simulink model "lo_values_test_v11"  (R2012b)
settings: Solver=ode45  StartTime=0.0  StopTime=100000  RelTol=1e-3
values from neighbouring files (symbols this model uses):
  Fs = 640e6    (= 640000000)    [filter_coefficients.m]    (also in filter_design.m; filter_design_getting_order.m)
undefined symbols (not defined in the file or in its folder): get, sided, Two
undefined symbols (not defined in the file): A_cos, A_sin, B_cos, B_sin, C_cos, C_sin, casper_coef, coef, D_cos, D_sin
libraries: xbsIndex_r4 x1768, dspsnks4 x10, casper_library_misc x9, xps_library x2, simulink x1
(part 6 of 17)

== system lo_values_test_v11/dec_fir2/fir_dbl_col38 ==
  real1 : Inport
  imag1 : Inport  Port=2
  real_back1 : Inport  Port=3
  imag_back1 : Inport  Port=4
  fir_dbl_tap1 : Subsystem  AncestorBlock=casper_library_downconverter/fir_dbl_tap  mask(fir_dbl_tap){factor=0.011867, add_latency=add_latency, mult_latency=mult_latency, coeff_bit_width=coeff_bit_width, coeff_bin_pt=coeff_bin_pt}
      mask prompts: add_latency "Add latency"; mult_latency "Mult latency"; coeff_bit_width "Coefficient bit width"; coeff_bin_pt "Coefficient binary point"
      mask init: same as lo_values_test_v11/dec_fir/fir_dbl_col1/fir_dbl_tap1
      mask Help: eval('xlWeb(''http://casper.berkeley.edu/wiki/Fir_dbl_tap'')')
  real_out1 : Outport
  imag_out1 : Outport  Port=2
  real_back_out1 : Outport  Port=3
  imag_back_out1 : Outport  Port=4
  real_sum : Outport  Port=5
  imag_sum : Outport  Port=6
  wires:
  real1/1 -> fir_dbl_tap1/1(a)
  imag1/1 -> fir_dbl_tap1/2(b)
  real_back1/1 -> fir_dbl_tap1/3(c)
  imag_back1/1 -> fir_dbl_tap1/4(d)
  fir_dbl_tap1/1(a_out) -> real_out1/1
  fir_dbl_tap1/2(b_out) -> imag_out1/1
  fir_dbl_tap1/3(c_out) -> real_back_out1/1
  fir_dbl_tap1/4(d_out) -> imag_back_out1/1
  fir_dbl_tap1/5(real) -> real_sum/1
  fir_dbl_tap1/6(imag) -> imag_sum/1

== system lo_values_test_v11/dec_fir2/fir_dbl_col39 ==
  real1 : Inport
  imag1 : Inport  Port=2
  real_back1 : Inport  Port=3
  imag_back1 : Inport  Port=4
  fir_dbl_tap1 : Subsystem  AncestorBlock=casper_library_downconverter/fir_dbl_tap  mask(fir_dbl_tap){factor=0.012277, add_latency=add_latency, mult_latency=mult_latency, coeff_bit_width=coeff_bit_width, coeff_bin_pt=coeff_bin_pt}
      mask prompts: add_latency "Add latency"; mult_latency "Mult latency"; coeff_bit_width "Coefficient bit width"; coeff_bin_pt "Coefficient binary point"
      mask init: same as lo_values_test_v11/dec_fir/fir_dbl_col1/fir_dbl_tap1
      mask Help: eval('xlWeb(''http://casper.berkeley.edu/wiki/Fir_dbl_tap'')')
  real_out1 : Outport
  imag_out1 : Outport  Port=2
  real_back_out1 : Outport  Port=3
  imag_back_out1 : Outport  Port=4
  real_sum : Outport  Port=5
  imag_sum : Outport  Port=6
  wires:
  real1/1 -> fir_dbl_tap1/1(a)
  imag1/1 -> fir_dbl_tap1/2(b)
  real_back1/1 -> fir_dbl_tap1/3(c)
  imag_back1/1 -> fir_dbl_tap1/4(d)
  fir_dbl_tap1/1(a_out) -> real_out1/1
  fir_dbl_tap1/2(b_out) -> imag_out1/1
  fir_dbl_tap1/3(c_out) -> real_back_out1/1
  fir_dbl_tap1/4(d_out) -> imag_back_out1/1
  fir_dbl_tap1/5(real) -> real_sum/1
  fir_dbl_tap1/6(imag) -> imag_sum/1

== system lo_values_test_v11/dec_fir2/fir_dbl_col4 ==
  real1 : Inport
  imag1 : Inport  Port=2
  real_back1 : Inport  Port=3
  imag_back1 : Inport  Port=4
  fir_dbl_tap1 : Subsystem  AncestorBlock=casper_library_downconverter/fir_dbl_tap  mask(fir_dbl_tap){factor=0.00035551, add_latency=add_latency, mult_latency=mult_latency, coeff_bit_width=coeff_bit_width, coeff_bin_pt=coeff_bin_pt}
      mask prompts: add_latency "Add latency"; mult_latency "Mult latency"; coeff_bit_width "Coefficient bit width"; coeff_bin_pt "Coefficient binary point"
      mask init: same as lo_values_test_v11/dec_fir/fir_dbl_col1/fir_dbl_tap1
      mask Help: eval('xlWeb(''http://casper.berkeley.edu/wiki/Fir_dbl_tap'')')
  real_out1 : Outport
  imag_out1 : Outport  Port=2
  real_back_out1 : Outport  Port=3
  imag_back_out1 : Outport  Port=4
  real_sum : Outport  Port=5
  imag_sum : Outport  Port=6
  wires:
  real1/1 -> fir_dbl_tap1/1(a)
  imag1/1 -> fir_dbl_tap1/2(b)
  real_back1/1 -> fir_dbl_tap1/3(c)
  imag_back1/1 -> fir_dbl_tap1/4(d)
  fir_dbl_tap1/1(a_out) -> real_out1/1
  fir_dbl_tap1/2(b_out) -> imag_out1/1
  fir_dbl_tap1/3(c_out) -> real_back_out1/1
  fir_dbl_tap1/4(d_out) -> imag_back_out1/1
  fir_dbl_tap1/5(real) -> real_sum/1
  fir_dbl_tap1/6(imag) -> imag_sum/1

== system lo_values_test_v11/dec_fir2/fir_dbl_col40 ==
  real1 : Inport
  imag1 : Inport  Port=2
  real_back1 : Inport  Port=3
  imag_back1 : Inport  Port=4
  fir_dbl_tap1 : Subsystem  AncestorBlock=casper_library_downconverter/fir_dbl_tap  mask(fir_dbl_tap){factor=0.012666, add_latency=add_latency, mult_latency=mult_latency, coeff_bit_width=coeff_bit_width, coeff_bin_pt=coeff_bin_pt}
      mask prompts: add_latency "Add latency"; mult_latency "Mult latency"; coeff_bit_width "Coefficient bit width"; coeff_bin_pt "Coefficient binary point"
      mask init: same as lo_values_test_v11/dec_fir/fir_dbl_col1/fir_dbl_tap1
      mask Help: eval('xlWeb(''http://casper.berkeley.edu/wiki/Fir_dbl_tap'')')
  real_out1 : Outport
  imag_out1 : Outport  Port=2
  real_back_out1 : Outport  Port=3
  imag_back_out1 : Outport  Port=4
  real_sum : Outport  Port=5
  imag_sum : Outport  Port=6
  wires:
  real1/1 -> fir_dbl_tap1/1(a)
  imag1/1 -> fir_dbl_tap1/2(b)
  real_back1/1 -> fir_dbl_tap1/3(c)
  imag_back1/1 -> fir_dbl_tap1/4(d)
  fir_dbl_tap1/1(a_out) -> real_out1/1
  fir_dbl_tap1/2(b_out) -> imag_out1/1
  fir_dbl_tap1/3(c_out) -> real_back_out1/1
  fir_dbl_tap1/4(d_out) -> imag_back_out1/1
  fir_dbl_tap1/5(real) -> real_sum/1
  fir_dbl_tap1/6(imag) -> imag_sum/1

== system lo_values_test_v11/dec_fir2/fir_dbl_col41 ==
  real1 : Inport
  imag1 : Inport  Port=2
  real_back1 : Inport  Port=3
  imag_back1 : Inport  Port=4
  fir_dbl_tap1 : Subsystem  AncestorBlock=casper_library_downconverter/fir_dbl_tap  mask(fir_dbl_tap){factor=0.013032, add_latency=add_latency, mult_latency=mult_latency, coeff_bit_width=coeff_bit_width, coeff_bin_pt=coeff_bin_pt}
      mask prompts: add_latency "Add latency"; mult_latency "Mult latency"; coeff_bit_width "Coefficient bit width"; coeff_bin_pt "Coefficient binary point"
      mask init: same as lo_values_test_v11/dec_fir/fir_dbl_col1/fir_dbl_tap1
      mask Help: eval('xlWeb(''http://casper.berkeley.edu/wiki/Fir_dbl_tap'')')
  real_out1 : Outport
  imag_out1 : Outport  Port=2
  real_back_out1 : Outport  Port=3
  imag_back_out1 : Outport  Port=4
  real_sum : Outport  Port=5
  imag_sum : Outport  Port=6
  wires:
  real1/1 -> fir_dbl_tap1/1(a)
  imag1/1 -> fir_dbl_tap1/2(b)
  real_back1/1 -> fir_dbl_tap1/3(c)
  imag_back1/1 -> fir_dbl_tap1/4(d)
  fir_dbl_tap1/1(a_out) -> real_out1/1
  fir_dbl_tap1/2(b_out) -> imag_out1/1
  fir_dbl_tap1/3(c_out) -> real_back_out1/1
  fir_dbl_tap1/4(d_out) -> imag_back_out1/1
  fir_dbl_tap1/5(real) -> real_sum/1
  fir_dbl_tap1/6(imag) -> imag_sum/1

== system lo_values_test_v11/dec_fir2/fir_dbl_col42 ==
  real1 : Inport
  imag1 : Inport  Port=2
  real_back1 : Inport  Port=3
  imag_back1 : Inport  Port=4
  fir_dbl_tap1 : Subsystem  AncestorBlock=casper_library_downconverter/fir_dbl_tap  mask(fir_dbl_tap){factor=0.013373, add_latency=add_latency, mult_latency=mult_latency, coeff_bit_width=coeff_bit_width, coeff_bin_pt=coeff_bin_pt}
      mask prompts: add_latency "Add latency"; mult_latency "Mult latency"; coeff_bit_width "Coefficient bit width"; coeff_bin_pt "Coefficient binary point"
      mask init: same as lo_values_test_v11/dec_fir/fir_dbl_col1/fir_dbl_tap1
      mask Help: eval('xlWeb(''http://casper.berkeley.edu/wiki/Fir_dbl_tap'')')
  real_out1 : Outport
  imag_out1 : Outport  Port=2
  real_back_out1 : Outport  Port=3
  imag_back_out1 : Outport  Port=4
  real_sum : Outport  Port=5
  imag_sum : Outport  Port=6
  wires:
  real1/1 -> fir_dbl_tap1/1(a)
  imag1/1 -> fir_dbl_tap1/2(b)
  real_back1/1 -> fir_dbl_tap1/3(c)
  imag_back1/1 -> fir_dbl_tap1/4(d)
  fir_dbl_tap1/1(a_out) -> real_out1/1
  fir_dbl_tap1/2(b_out) -> imag_out1/1
  fir_dbl_tap1/3(c_out) -> real_back_out1/1
  fir_dbl_tap1/4(d_out) -> imag_back_out1/1
  fir_dbl_tap1/5(real) -> real_sum/1
  fir_dbl_tap1/6(imag) -> imag_sum/1

== system lo_values_test_v11/dec_fir2/fir_dbl_col43 ==
  real1 : Inport
  imag1 : Inport  Port=2
  real_back1 : Inport  Port=3
  imag_back1 : Inport  Port=4
  fir_dbl_tap1 : Subsystem  AncestorBlock=casper_library_downconverter/fir_dbl_tap  mask(fir_dbl_tap){factor=0.013686, add_latency=add_latency, mult_latency=mult_latency, coeff_bit_width=coeff_bit_width, coeff_bin_pt=coeff_bin_pt}
      mask prompts: add_latency "Add latency"; mult_latency "Mult latency"; coeff_bit_width "Coefficient bit width"; coeff_bin_pt "Coefficient binary point"
      mask init: same as lo_values_test_v11/dec_fir/fir_dbl_col1/fir_dbl_tap1
      mask Help: eval('xlWeb(''http://casper.berkeley.edu/wiki/Fir_dbl_tap'')')
  real_out1 : Outport
  imag_out1 : Outport  Port=2
  real_back_out1 : Outport  Port=3
  imag_back_out1 : Outport  Port=4
  real_sum : Outport  Port=5
  imag_sum : Outport  Port=6
  wires:
  real1/1 -> fir_dbl_tap1/1(a)
  imag1/1 -> fir_dbl_tap1/2(b)
  real_back1/1 -> fir_dbl_tap1/3(c)
  imag_back1/1 -> fir_dbl_tap1/4(d)
  fir_dbl_tap1/1(a_out) -> real_out1/1
  fir_dbl_tap1/2(b_out) -> imag_out1/1
  fir_dbl_tap1/3(c_out) -> real_back_out1/1
  fir_dbl_tap1/4(d_out) -> imag_back_out1/1
  fir_dbl_tap1/5(real) -> real_sum/1
  fir_dbl_tap1/6(imag) -> imag_sum/1

== system lo_values_test_v11/dec_fir2/fir_dbl_col44 ==
  real1 : Inport
  imag1 : Inport  Port=2
  real_back1 : Inport  Port=3
  imag_back1 : Inport  Port=4
  fir_dbl_tap1 : Subsystem  AncestorBlock=casper_library_downconverter/fir_dbl_tap  mask(fir_dbl_tap){factor=0.01397, add_latency=add_latency, mult_latency=mult_latency, coeff_bit_width=coeff_bit_width, coeff_bin_pt=coeff_bin_pt}
      mask prompts: add_latency "Add latency"; mult_latency "Mult latency"; coeff_bit_width "Coefficient bit width"; coeff_bin_pt "Coefficient binary point"
      mask init: same as lo_values_test_v11/dec_fir/fir_dbl_col1/fir_dbl_tap1
      mask Help: eval('xlWeb(''http://casper.berkeley.edu/wiki/Fir_dbl_tap'')')
  real_out1 : Outport
  imag_out1 : Outport  Port=2
  real_back_out1 : Outport  Port=3
  imag_back_out1 : Outport  Port=4
  real_sum : Outport  Port=5
  imag_sum : Outport  Port=6
  wires:
  real1/1 -> fir_dbl_tap1/1(a)
  imag1/1 -> fir_dbl_tap1/2(b)
  real_back1/1 -> fir_dbl_tap1/3(c)
  imag_back1/1 -> fir_dbl_tap1/4(d)
  fir_dbl_tap1/1(a_out) -> real_out1/1
  fir_dbl_tap1/2(b_out) -> imag_out1/1
  fir_dbl_tap1/3(c_out) -> real_back_out1/1
  fir_dbl_tap1/4(d_out) -> imag_back_out1/1
  fir_dbl_tap1/5(real) -> real_sum/1
  fir_dbl_tap1/6(imag) -> imag_sum/1

== system lo_values_test_v11/dec_fir2/fir_dbl_col45 ==
  real1 : Inport
  imag1 : Inport  Port=2
  real_back1 : Inport  Port=3
  imag_back1 : Inport  Port=4
  fir_dbl_tap1 : Subsystem  AncestorBlock=casper_library_downconverter/fir_dbl_tap  mask(fir_dbl_tap){factor=0.014223, add_latency=add_latency, mult_latency=mult_latency, coeff_bit_width=coeff_bit_width, coeff_bin_pt=coeff_bin_pt}
      mask prompts: add_latency "Add latency"; mult_latency "Mult latency"; coeff_bit_width "Coefficient bit width"; coeff_bin_pt "Coefficient binary point"
      mask init: same as lo_values_test_v11/dec_fir/fir_dbl_col1/fir_dbl_tap1
      mask Help: eval('xlWeb(''http://casper.berkeley.edu/wiki/Fir_dbl_tap'')')
  real_out1 : Outport
  imag_out1 : Outport  Port=2
  real_back_out1 : Outport  Port=3
  imag_back_out1 : Outport  Port=4
  real_sum : Outport  Port=5
  imag_sum : Outport  Port=6
  wires:
  real1/1 -> fir_dbl_tap1/1(a)
  imag1/1 -> fir_dbl_tap1/2(b)
  real_back1/1 -> fir_dbl_tap1/3(c)
  imag_back1/1 -> fir_dbl_tap1/4(d)
  fir_dbl_tap1/1(a_out) -> real_out1/1
  fir_dbl_tap1/2(b_out) -> imag_out1/1
  fir_dbl_tap1/3(c_out) -> real_back_out1/1
  fir_dbl_tap1/4(d_out) -> imag_back_out1/1
  fir_dbl_tap1/5(real) -> real_sum/1
  fir_dbl_tap1/6(imag) -> imag_sum/1

== system lo_values_test_v11/dec_fir2/fir_dbl_col46 ==
  real1 : Inport
  imag1 : Inport  Port=2
  real_back1 : Inport  Port=3
  imag_back1 : Inport  Port=4
  fir_dbl_tap1 : Subsystem  AncestorBlock=casper_library_downconverter/fir_dbl_tap  mask(fir_dbl_tap){factor=0.014442, add_latency=add_latency, mult_latency=mult_latency, coeff_bit_width=coeff_bit_width, coeff_bin_pt=coeff_bin_pt}
      mask prompts: add_latency "Add latency"; mult_latency "Mult latency"; coeff_bit_width "Coefficient bit width"; coeff_bin_pt "Coefficient binary point"
      mask init: same as lo_values_test_v11/dec_fir/fir_dbl_col1/fir_dbl_tap1
      mask Help: eval('xlWeb(''http://casper.berkeley.edu/wiki/Fir_dbl_tap'')')
  real_out1 : Outport
  imag_out1 : Outport  Port=2
  real_back_out1 : Outport  Port=3
  imag_back_out1 : Outport  Port=4
  real_sum : Outport  Port=5
  imag_sum : Outport  Port=6
  wires:
  real1/1 -> fir_dbl_tap1/1(a)
  imag1/1 -> fir_dbl_tap1/2(b)
  real_back1/1 -> fir_dbl_tap1/3(c)
  imag_back1/1 -> fir_dbl_tap1/4(d)
  fir_dbl_tap1/1(a_out) -> real_out1/1
  fir_dbl_tap1/2(b_out) -> imag_out1/1
  fir_dbl_tap1/3(c_out) -> real_back_out1/1
  fir_dbl_tap1/4(d_out) -> imag_back_out1/1
  fir_dbl_tap1/5(real) -> real_sum/1
  fir_dbl_tap1/6(imag) -> imag_sum/1

== system lo_values_test_v11/dec_fir2/fir_dbl_col47 ==
  real1 : Inport
  imag1 : Inport  Port=2
  real_back1 : Inport  Port=3
  imag_back1 : Inport  Port=4
  fir_dbl_tap1 : Subsystem  AncestorBlock=casper_library_downconverter/fir_dbl_tap  mask(fir_dbl_tap){factor=0.014628, add_latency=add_latency, mult_latency=mult_latency, coeff_bit_width=coeff_bit_width, coeff_bin_pt=coeff_bin_pt}
      mask prompts: add_latency "Add latency"; mult_latency "Mult latency"; coeff_bit_width "Coefficient bit width"; coeff_bin_pt "Coefficient binary point"
      mask init: same as lo_values_test_v11/dec_fir/fir_dbl_col1/fir_dbl_tap1
      mask Help: eval('xlWeb(''http://casper.berkeley.edu/wiki/Fir_dbl_tap'')')
  real_out1 : Outport
  imag_out1 : Outport  Port=2
  real_back_out1 : Outport  Port=3
  imag_back_out1 : Outport  Port=4
  real_sum : Outport  Port=5
  imag_sum : Outport  Port=6
  wires:
  real1/1 -> fir_dbl_tap1/1(a)
  imag1/1 -> fir_dbl_tap1/2(b)
  real_back1/1 -> fir_dbl_tap1/3(c)
  imag_back1/1 -> fir_dbl_tap1/4(d)
  fir_dbl_tap1/1(a_out) -> real_out1/1
  fir_dbl_tap1/2(b_out) -> imag_out1/1
  fir_dbl_tap1/3(c_out) -> real_back_out1/1
  fir_dbl_tap1/4(d_out) -> imag_back_out1/1
  fir_dbl_tap1/5(real) -> real_sum/1
  fir_dbl_tap1/6(imag) -> imag_sum/1

== system lo_values_test_v11/dec_fir2/fir_dbl_col48 ==
  real1 : Inport
  imag1 : Inport  Port=2
  real_back1 : Inport  Port=3
  imag_back1 : Inport  Port=4
  fir_dbl_tap1 : Subsystem  AncestorBlock=casper_library_downconverter/fir_dbl_tap  mask(fir_dbl_tap){factor=0.014778, add_latency=add_latency, mult_latency=mult_latency, coeff_bit_width=coeff_bit_width, coeff_bin_pt=coeff_bin_pt}
      mask prompts: add_latency "Add latency"; mult_latency "Mult latency"; coeff_bit_width "Coefficient bit width"; coeff_bin_pt "Coefficient binary point"
      mask init: same as lo_values_test_v11/dec_fir/fir_dbl_col1/fir_dbl_tap1
      mask Help: eval('xlWeb(''http://casper.berkeley.edu/wiki/Fir_dbl_tap'')')
  real_out1 : Outport
  imag_out1 : Outport  Port=2
  real_back_out1 : Outport  Port=3
  imag_back_out1 : Outport  Port=4
  real_sum : Outport  Port=5
  imag_sum : Outport  Port=6
  wires:
  real1/1 -> fir_dbl_tap1/1(a)
  imag1/1 -> fir_dbl_tap1/2(b)
  real_back1/1 -> fir_dbl_tap1/3(c)
  imag_back1/1 -> fir_dbl_tap1/4(d)
  fir_dbl_tap1/1(a_out) -> real_out1/1
  fir_dbl_tap1/2(b_out) -> imag_out1/1
  fir_dbl_tap1/3(c_out) -> real_back_out1/1
  fir_dbl_tap1/4(d_out) -> imag_back_out1/1
  fir_dbl_tap1/5(real) -> real_sum/1
  fir_dbl_tap1/6(imag) -> imag_sum/1

== system lo_values_test_v11/dec_fir2/fir_dbl_col49 ==
  real1 : Inport
  imag1 : Inport  Port=2
  real_back1 : Inport  Port=3
  imag_back1 : Inport  Port=4
  fir_dbl_tap1 : Subsystem  AncestorBlock=casper_library_downconverter/fir_dbl_tap  mask(fir_dbl_tap){factor=0.014891, add_latency=add_latency, mult_latency=mult_latency, coeff_bit_width=coeff_bit_width, coeff_bin_pt=coeff_bin_pt}
      mask prompts: add_latency "Add latency"; mult_latency "Mult latency"; coeff_bit_width "Coefficient bit width"; coeff_bin_pt "Coefficient binary point"
      mask init: same as lo_values_test_v11/dec_fir/fir_dbl_col1/fir_dbl_tap1
      mask Help: eval('xlWeb(''http://casper.berkeley.edu/wiki/Fir_dbl_tap'')')
  real_out1 : Outport
  imag_out1 : Outport  Port=2
  real_back_out1 : Outport  Port=3
  imag_back_out1 : Outport  Port=4
  real_sum : Outport  Port=5
  imag_sum : Outport  Port=6
  wires:
  real1/1 -> fir_dbl_tap1/1(a)
  imag1/1 -> fir_dbl_tap1/2(b)
  real_back1/1 -> fir_dbl_tap1/3(c)
  imag_back1/1 -> fir_dbl_tap1/4(d)
  fir_dbl_tap1/1(a_out) -> real_out1/1
  fir_dbl_tap1/2(b_out) -> imag_out1/1
  fir_dbl_tap1/3(c_out) -> real_back_out1/1
  fir_dbl_tap1/4(d_out) -> imag_back_out1/1
  fir_dbl_tap1/5(real) -> real_sum/1
  fir_dbl_tap1/6(imag) -> imag_sum/1

== system lo_values_test_v11/dec_fir2/fir_dbl_col5 ==
  real1 : Inport
  imag1 : Inport  Port=2
  real_back1 : Inport  Port=3
  imag_back1 : Inport  Port=4
  fir_dbl_tap1 : Subsystem  AncestorBlock=casper_library_downconverter/fir_dbl_tap  mask(fir_dbl_tap){factor=0.00044384, add_latency=add_latency, mult_latency=mult_latency, coeff_bit_width=coeff_bit_width, coeff_bin_pt=coeff_bin_pt}
      mask prompts: add_latency "Add latency"; mult_latency "Mult latency"; coeff_bit_width "Coefficient bit width"; coeff_bin_pt "Coefficient binary point"
      mask init: same as lo_values_test_v11/dec_fir/fir_dbl_col1/fir_dbl_tap1
      mask Help: eval('xlWeb(''http://casper.berkeley.edu/wiki/Fir_dbl_tap'')')
  real_out1 : Outport
  imag_out1 : Outport  Port=2
  real_back_out1 : Outport  Port=3
  imag_back_out1 : Outport  Port=4
  real_sum : Outport  Port=5
  imag_sum : Outport  Port=6
  wires:
  real1/1 -> fir_dbl_tap1/1(a)
  imag1/1 -> fir_dbl_tap1/2(b)
  real_back1/1 -> fir_dbl_tap1/3(c)
  imag_back1/1 -> fir_dbl_tap1/4(d)
  fir_dbl_tap1/1(a_out) -> real_out1/1
  fir_dbl_tap1/2(b_out) -> imag_out1/1
  fir_dbl_tap1/3(c_out) -> real_back_out1/1
  fir_dbl_tap1/4(d_out) -> imag_back_out1/1
  fir_dbl_tap1/5(real) -> real_sum/1
  fir_dbl_tap1/6(imag) -> imag_sum/1

== system lo_values_test_v11/dec_fir2/fir_dbl_col50 ==
  real1 : Inport
  imag1 : Inport  Port=2
  real_back1 : Inport  Port=3
  imag_back1 : Inport  Port=4
  fir_dbl_tap1 : Subsystem  AncestorBlock=casper_library_downconverter/fir_dbl_tap  mask(fir_dbl_tap){factor=0.014967, add_latency=add_latency, mult_latency=mult_latency, coeff_bit_width=coeff_bit_width, coeff_bin_pt=coeff_bin_pt}
      mask prompts: add_latency "Add latency"; mult_latency "Mult latency"; coeff_bit_width "Coefficient bit width"; coeff_bin_pt "Coefficient binary point"
      mask init: same as lo_values_test_v11/dec_fir/fir_dbl_col1/fir_dbl_tap1
      mask Help: eval('xlWeb(''http://casper.berkeley.edu/wiki/Fir_dbl_tap'')')
  real_out1 : Outport
  imag_out1 : Outport  Port=2
  real_back_out1 : Outport  Port=3
  imag_back_out1 : Outport  Port=4
  real_sum : Outport  Port=5
  imag_sum : Outport  Port=6
  wires:
  real1/1 -> fir_dbl_tap1/1(a)
  imag1/1 -> fir_dbl_tap1/2(b)
  real_back1/1 -> fir_dbl_tap1/3(c)
  imag_back1/1 -> fir_dbl_tap1/4(d)
  fir_dbl_tap1/1(a_out) -> real_out1/1
  fir_dbl_tap1/2(b_out) -> imag_out1/1
  fir_dbl_tap1/3(c_out) -> real_back_out1/1
  fir_dbl_tap1/4(d_out) -> imag_back_out1/1
  fir_dbl_tap1/5(real) -> real_sum/1
  fir_dbl_tap1/6(imag) -> imag_sum/1

== system lo_values_test_v11/dec_fir2/fir_dbl_col51 ==
  real1 : Inport
  imag1 : Inport  Port=2
  real_back1 : Inport  Port=3
  imag_back1 : Inport  Port=4
  fir_dbl_tap1 : Subsystem  AncestorBlock=casper_library_downconverter/fir_dbl_tap  mask(fir_dbl_tap){factor=0.015005, add_latency=add_latency, mult_latency=mult_latency, coeff_bit_width=coeff_bit_width, coeff_bin_pt=coeff_bin_pt}
      mask prompts: add_latency "Add latency"; mult_latency "Mult latency"; coeff_bit_width "Coefficient bit width"; coeff_bin_pt "Coefficient binary point"
      mask init: same as lo_values_test_v11/dec_fir/fir_dbl_col1/fir_dbl_tap1
      mask Help: eval('xlWeb(''http://casper.berkeley.edu/wiki/Fir_dbl_tap'')')
  real_out1 : Outport
  imag_out1 : Outport  Port=2
  real_back_out1 : Outport  Port=3
  imag_back_out1 : Outport  Port=4
  real_sum : Outport  Port=5
  imag_sum : Outport  Port=6
  wires:
  real1/1 -> fir_dbl_tap1/1(a)
  imag1/1 -> fir_dbl_tap1/2(b)
  real_back1/1 -> fir_dbl_tap1/3(c)
  imag_back1/1 -> fir_dbl_tap1/4(d)
  fir_dbl_tap1/1(a_out) -> real_out1/1
  fir_dbl_tap1/2(b_out) -> imag_out1/1
  fir_dbl_tap1/3(c_out) -> real_back_out1/1
  fir_dbl_tap1/4(d_out) -> imag_back_out1/1
  fir_dbl_tap1/5(real) -> real_sum/1
  fir_dbl_tap1/6(imag) -> imag_sum/1

== system lo_values_test_v11/dec_fir2/fir_dbl_col6 ==
  real1 : Inport
  imag1 : Inport  Port=2
  real_back1 : Inport  Port=3
  imag_back1 : Inport  Port=4
  fir_dbl_tap1 : Subsystem  AncestorBlock=casper_library_downconverter/fir_dbl_tap  mask(fir_dbl_tap){factor=0.00054573, add_latency=add_latency, mult_latency=mult_latency, coeff_bit_width=coeff_bit_width, coeff_bin_pt=coeff_bin_pt}
      mask prompts: add_latency "Add latency"; mult_latency "Mult latency"; coeff_bit_width "Coefficient bit width"; coeff_bin_pt "Coefficient binary point"
      mask init: same as lo_values_test_v11/dec_fir/fir_dbl_col1/fir_dbl_tap1
      mask Help: eval('xlWeb(''http://casper.berkeley.edu/wiki/Fir_dbl_tap'')')
  real_out1 : Outport
  imag_out1 : Outport  Port=2
  real_back_out1 : Outport  Port=3
  imag_back_out1 : Outport  Port=4
  real_sum : Outport  Port=5
  imag_sum : Outport  Port=6
  wires:
  real1/1 -> fir_dbl_tap1/1(a)
  imag1/1 -> fir_dbl_tap1/2(b)
  real_back1/1 -> fir_dbl_tap1/3(c)
  imag_back1/1 -> fir_dbl_tap1/4(d)
  fir_dbl_tap1/1(a_out) -> real_out1/1
  fir_dbl_tap1/2(b_out) -> imag_out1/1
  fir_dbl_tap1/3(c_out) -> real_back_out1/1
  fir_dbl_tap1/4(d_out) -> imag_back_out1/1
  fir_dbl_tap1/5(real) -> real_sum/1
  fir_dbl_tap1/6(imag) -> imag_sum/1

== system lo_values_test_v11/dec_fir2/fir_dbl_col7 ==
  real1 : Inport
  imag1 : Inport  Port=2
  real_back1 : Inport  Port=3
  imag_back1 : Inport  Port=4
  fir_dbl_tap1 : Subsystem  AncestorBlock=casper_library_downconverter/fir_dbl_tap  mask(fir_dbl_tap){factor=0.00066171, add_latency=add_latency, mult_latency=mult_latency, coeff_bit_width=coeff_bit_width, coeff_bin_pt=coeff_bin_pt}
      mask prompts: add_latency "Add latency"; mult_latency "Mult latency"; coeff_bit_width "Coefficient bit width"; coeff_bin_pt "Coefficient binary point"
      mask init: same as lo_values_test_v11/dec_fir/fir_dbl_col1/fir_dbl_tap1
      mask Help: eval('xlWeb(''http://casper.berkeley.edu/wiki/Fir_dbl_tap'')')
  real_out1 : Outport
  imag_out1 : Outport  Port=2
  real_back_out1 : Outport  Port=3
  imag_back_out1 : Outport  Port=4
  real_sum : Outport  Port=5
  imag_sum : Outport  Port=6
  wires:
  real1/1 -> fir_dbl_tap1/1(a)
  imag1/1 -> fir_dbl_tap1/2(b)
  real_back1/1 -> fir_dbl_tap1/3(c)
  imag_back1/1 -> fir_dbl_tap1/4(d)
  fir_dbl_tap1/1(a_out) -> real_out1/1
  fir_dbl_tap1/2(b_out) -> imag_out1/1
  fir_dbl_tap1/3(c_out) -> real_back_out1/1
  fir_dbl_tap1/4(d_out) -> imag_back_out1/1
  fir_dbl_tap1/5(real) -> real_sum/1
  fir_dbl_tap1/6(imag) -> imag_sum/1

== system lo_values_test_v11/dec_fir2/fir_dbl_col8 ==
  real1 : Inport
  imag1 : Inport  Port=2
  real_back1 : Inport  Port=3
  imag_back1 : Inport  Port=4
  fir_dbl_tap1 : Subsystem  AncestorBlock=casper_library_downconverter/fir_dbl_tap  mask(fir_dbl_tap){factor=0.00079278, add_latency=add_latency, mult_latency=mult_latency, coeff_bit_width=coeff_bit_width, coeff_bin_pt=coeff_bin_pt}
      mask prompts: add_latency "Add latency"; mult_latency "Mult latency"; coeff_bit_width "Coefficient bit width"; coeff_bin_pt "Coefficient binary point"
      mask init: same as lo_values_test_v11/dec_fir/fir_dbl_col1/fir_dbl_tap1
      mask Help: eval('xlWeb(''http://casper.berkeley.edu/wiki/Fir_dbl_tap'')')
  real_out1 : Outport
  imag_out1 : Outport  Port=2
  real_back_out1 : Outport  Port=3
  imag_back_out1 : Outport  Port=4
  real_sum : Outport  Port=5
  imag_sum : Outport  Port=6
  wires:
  real1/1 -> fir_dbl_tap1/1(a)
  imag1/1 -> fir_dbl_tap1/2(b)
  real_back1/1 -> fir_dbl_tap1/3(c)
  imag_back1/1 -> fir_dbl_tap1/4(d)
  fir_dbl_tap1/1(a_out) -> real_out1/1
  fir_dbl_tap1/2(b_out) -> imag_out1/1
  fir_dbl_tap1/3(c_out) -> real_back_out1/1
  fir_dbl_tap1/4(d_out) -> imag_back_out1/1
  fir_dbl_tap1/5(real) -> real_sum/1
  fir_dbl_tap1/6(imag) -> imag_sum/1

== system lo_values_test_v11/dec_fir2/fir_dbl_col9 ==
  real1 : Inport
  imag1 : Inport  Port=2
  real_back1 : Inport  Port=3
  imag_back1 : Inport  Port=4
  fir_dbl_tap1 : Subsystem  AncestorBlock=casper_library_downconverter/fir_dbl_tap  mask(fir_dbl_tap){factor=0.00093982, add_latency=add_latency, mult_latency=mult_latency, coeff_bit_width=coeff_bit_width, coeff_bin_pt=coeff_bin_pt}
      mask prompts: add_latency "Add latency"; mult_latency "Mult latency"; coeff_bit_width "Coefficient bit width"; coeff_bin_pt "Coefficient binary point"
      mask init: same as lo_values_test_v11/dec_fir/fir_dbl_col1/fir_dbl_tap1
      mask Help: eval('xlWeb(''http://casper.berkeley.edu/wiki/Fir_dbl_tap'')')
  real_out1 : Outport
  imag_out1 : Outport  Port=2
  real_back_out1 : Outport  Port=3
  imag_back_out1 : Outport  Port=4
  real_sum : Outport  Port=5
  imag_sum : Outport  Port=6
  wires:
  real1/1 -> fir_dbl_tap1/1(a)
  imag1/1 -> fir_dbl_tap1/2(b)
  real_back1/1 -> fir_dbl_tap1/3(c)
  imag_back1/1 -> fir_dbl_tap1/4(d)
  fir_dbl_tap1/1(a_out) -> real_out1/1
  fir_dbl_tap1/2(b_out) -> imag_out1/1
  fir_dbl_tap1/3(c_out) -> real_back_out1/1
  fir_dbl_tap1/4(d_out) -> imag_back_out1/1
  fir_dbl_tap1/5(real) -> real_sum/1
  fir_dbl_tap1/6(imag) -> imag_sum/1

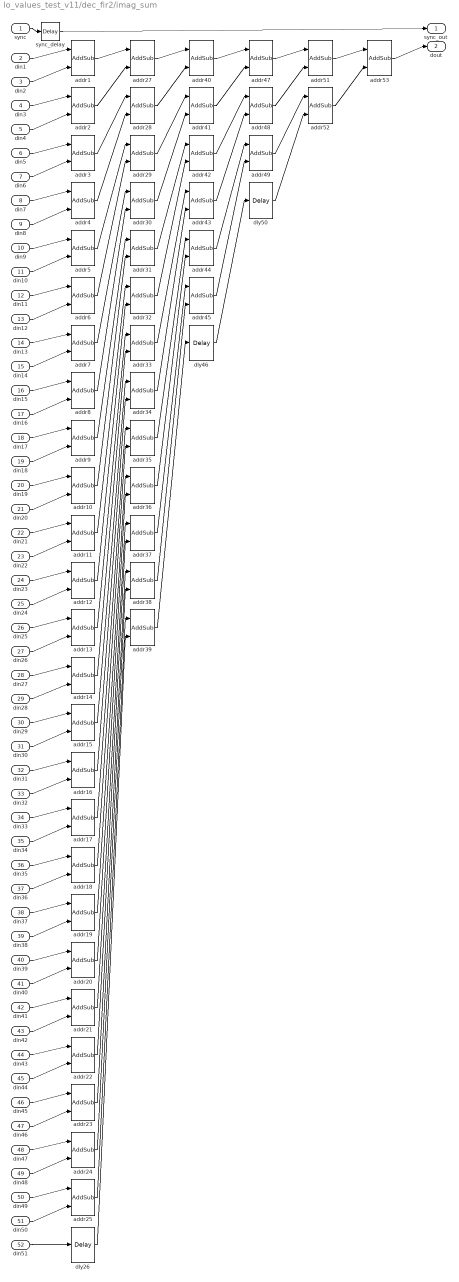
== system lo_values_test_v11/dec_fir2/imag_sum ==
  sync : Inport
  din1 : Inport  Port=2
  din2 : Inport  Port=3
  din3 : Inport  Port=4
  din4 : Inport  Port=5
  din5 : Inport  Port=6
  din6 : Inport  Port=7
  din7 : Inport  Port=8
  din8 : Inport  Port=9
  din9 : Inport  Port=10
  din10 : Inport  Port=11
  din11 : Inport  Port=12
  din12 : Inport  Port=13
  din13 : Inport  Port=14
  din14 : Inport  Port=15
  din15 : Inport  Port=16
  din16 : Inport  Port=17
  din17 : Inport  Port=18
  din18 : Inport  Port=19
  din19 : Inport  Port=20
  din20 : Inport  Port=21
  din21 : Inport  Port=22
  din22 : Inport  Port=23
  din23 : Inport  Port=24
  din24 : Inport  Port=25
  din25 : Inport  Port=26
  din26 : Inport  Port=27
  din27 : Inport  Port=28
  din28 : Inport  Port=29
  din29 : Inport  Port=30
  din30 : Inport  Port=31
  din31 : Inport  Port=32
  din32 : Inport  Port=33
  din33 : Inport  Port=34
  din34 : Inport  Port=35
  din35 : Inport  Port=36
  din36 : Inport  Port=37
  din37 : Inport  Port=38
  din38 : Inport  Port=39
  din39 : Inport  Port=40
  din40 : Inport  Port=41
  din41 : Inport  Port=42
  din42 : Inport  Port=43
  din43 : Inport  Port=44
  din44 : Inport  Port=45
  din45 : Inport  Port=46
  din46 : Inport  Port=47
  din47 : Inport  Port=48
  din48 : Inport  Port=49
  din49 : Inport  Port=50
  din50 : Inport  Port=51
  din51 : Inport  Port=52
  addr{1..25} (25 alike) : xbsIndex_r4/AddSub  mode=Addition  use_carryin=off  use_carryout=off  en=off  latency=1  precision=Full  arith_type=Unsigned  n_bits=16  bin_pt=14  quantization=Truncate  overflow=Wrap  dbl_ovrd=off  use_behavioral_HDL=on  hw_selection=DSP48  pipelined=on  use_rpm=on  block_type=addsub
  addr{27..45,47..49,51..53} (25 alike) : xbsIndex_r4/AddSub  mode=Addition  use_carryin=off  use_carryout=off  en=off  latency=1  precision=Full  arith_type=Unsigned  n_bits=16  bin_pt=14  quantization=Truncate  overflow=Wrap  dbl_ovrd=off  use_behavioral_HDL=off  hw_selection=DSP48  pipelined=on  use_rpm=on  block_type=addsub
  dly26 : xbsIndex_r4/Delay  rst=off  infoeditControl=Selection of Reset will increase slice count due to use of real FFs and instead of SRLs  en=off  latency=1  dbl_ovrd=off  reg_retiming=on  block_type=delay
  dly46 : xbsIndex_r4/Delay  rst=off  infoeditControl=Selection of Reset will increase slice count due to use of real FFs and instead of SRLs  en=off  latency=1  dbl_ovrd=off  reg_retiming=on  block_type=delay
  dly50 : xbsIndex_r4/Delay  rst=off  infoeditControl=Selection of Reset will increase slice count due to use of real FFs and instead of SRLs  en=off  latency=1  dbl_ovrd=off  reg_retiming=on  block_type=delay
  sync_delay : xbsIndex_r4/Delay  rst=off  infoeditControl=Selection of Reset will increase slice count due to use of real FFs and instead of SRLs  en=off  latency=6  dbl_ovrd=off  reg_retiming=on  block_type=delay
      settings: block_version=11.4
  sync_out : Outport
  dout : Outport  Port=2
  wires:
  sync/1 -> sync_delay/1
  sync_delay/1 -> sync_out/1
  din1/1 -> addr1/1
  din2/1 -> addr1/2
  din3/1 -> addr2/1
  din4/1 -> addr2/2
  din5/1 -> addr3/1
  din6/1 -> addr3/2
  din7/1 -> addr4/1
  din8/1 -> addr4/2
  din9/1 -> addr5/1
  din10/1 -> addr5/2
  din11/1 -> addr6/1
  din12/1 -> addr6/2
  din13/1 -> addr7/1
  din14/1 -> addr7/2
  din15/1 -> addr8/1
  din16/1 -> addr8/2
  din17/1 -> addr9/1
  din18/1 -> addr9/2
  din19/1 -> addr10/1
  din20/1 -> addr10/2
  din21/1 -> addr11/1
  din22/1 -> addr11/2
  din23/1 -> addr12/1
  din24/1 -> addr12/2
  din25/1 -> addr13/1
  din26/1 -> addr13/2
  din27/1 -> addr14/1
  din28/1 -> addr14/2
  din29/1 -> addr15/1
  din30/1 -> addr15/2
  din31/1 -> addr16/1
  din32/1 -> addr16/2
  din33/1 -> addr17/1
  din34/1 -> addr17/2
  din35/1 -> addr18/1
  din36/1 -> addr18/2
  din37/1 -> addr19/1
  din38/1 -> addr19/2
  din39/1 -> addr20/1
  din40/1 -> addr20/2
  din41/1 -> addr21/1
  din42/1 -> addr21/2
  din43/1 -> addr22/1
  din44/1 -> addr22/2
  din45/1 -> addr23/1
  din46/1 -> addr23/2
  din47/1 -> addr24/1
  din48/1 -> addr24/2
  din49/1 -> addr25/1
  din50/1 -> addr25/2
  din51/1 -> dly26/1
  addr1/1 -> addr27/1
  addr2/1 -> addr27/2
  addr3/1 -> addr28/1
  addr4/1 -> addr28/2
  addr5/1 -> addr29/1
  addr6/1 -> addr29/2
  addr7/1 -> addr30/1
  addr8/1 -> addr30/2
  addr9/1 -> addr31/1
  addr10/1 -> addr31/2
  addr11/1 -> addr32/1
  addr12/1 -> addr32/2
  addr13/1 -> addr33/1
  addr14/1 -> addr33/2
  addr15/1 -> addr34/1
  addr16/1 -> addr34/2
  addr17/1 -> addr35/1
  addr18/1 -> addr35/2
  addr19/1 -> addr36/1
  addr20/1 -> addr36/2
  addr21/1 -> addr37/1
  addr22/1 -> addr37/2
  addr23/1 -> addr38/1
  addr24/1 -> addr38/2
  addr25/1 -> addr39/1
  dly26/1 -> addr39/2
  addr27/1 -> addr40/1
  addr28/1 -> addr40/2
  addr29/1 -> addr41/1
  addr30/1 -> addr41/2
  addr31/1 -> addr42/1
  addr32/1 -> addr42/2
  addr33/1 -> addr43/1
  addr34/1 -> addr43/2
  addr35/1 -> addr44/1
  addr36/1 -> addr44/2
  addr37/1 -> addr45/1
  addr38/1 -> addr45/2
  addr39/1 -> dly46/1
  addr40/1 -> addr47/1
  addr41/1 -> addr47/2
  addr42/1 -> addr48/1
  addr43/1 -> addr48/2
  addr44/1 -> addr49/1
  addr45/1 -> addr49/2
  dly46/1 -> dly50/1
  addr47/1 -> addr51/1
  addr48/1 -> addr51/2
  addr49/1 -> addr52/1
  dly50/1 -> addr52/2
  addr51/1 -> addr53/1
  addr52/1 -> addr53/2
  addr53/1 -> dout/1

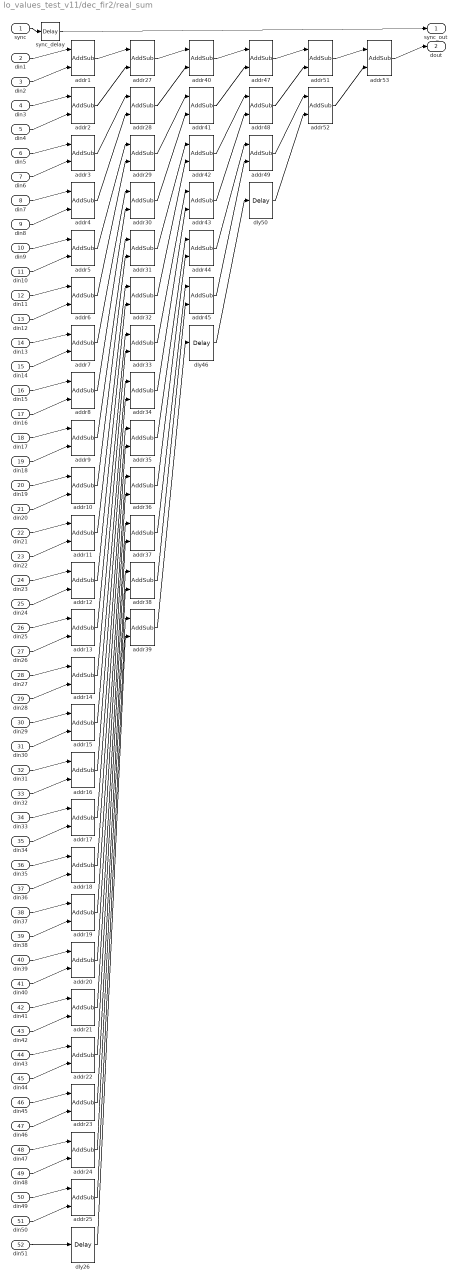
== system lo_values_test_v11/dec_fir2/real_sum ==
  sync : Inport
  din1 : Inport  Port=2
  din2 : Inport  Port=3
  din3 : Inport  Port=4
  din4 : Inport  Port=5
  din5 : Inport  Port=6
  din6 : Inport  Port=7
  din7 : Inport  Port=8
  din8 : Inport  Port=9
  din9 : Inport  Port=10
  din10 : Inport  Port=11
  din11 : Inport  Port=12
  din12 : Inport  Port=13
  din13 : Inport  Port=14
  din14 : Inport  Port=15
  din15 : Inport  Port=16
  din16 : Inport  Port=17
  din17 : Inport  Port=18
  din18 : Inport  Port=19
  din19 : Inport  Port=20
  din20 : Inport  Port=21
  din21 : Inport  Port=22
  din22 : Inport  Port=23
  din23 : Inport  Port=24
  din24 : Inport  Port=25
  din25 : Inport  Port=26
  din26 : Inport  Port=27
  din27 : Inport  Port=28
  din28 : Inport  Port=29
  din29 : Inport  Port=30
  din30 : Inport  Port=31
  din31 : Inport  Port=32
  din32 : Inport  Port=33
  din33 : Inport  Port=34
  din34 : Inport  Port=35
  din35 : Inport  Port=36
  din36 : Inport  Port=37
  din37 : Inport  Port=38
  din38 : Inport  Port=39
  din39 : Inport  Port=40
  din40 : Inport  Port=41
  din41 : Inport  Port=42
  din42 : Inport  Port=43
  din43 : Inport  Port=44
  din44 : Inport  Port=45
  din45 : Inport  Port=46
  din46 : Inport  Port=47
  din47 : Inport  Port=48
  din48 : Inport  Port=49
  din49 : Inport  Port=50
  din50 : Inport  Port=51
  din51 : Inport  Port=52
  addr{1..25} (25 alike) : xbsIndex_r4/AddSub  mode=Addition  use_carryin=off  use_carryout=off  en=off  latency=1  precision=Full  arith_type=Unsigned  n_bits=16  bin_pt=14  quantization=Truncate  overflow=Wrap  dbl_ovrd=off  use_behavioral_HDL=on  hw_selection=DSP48  pipelined=on  use_rpm=on  block_type=addsub
  addr{27..45,47..49,51..53} (25 alike) : xbsIndex_r4/AddSub  mode=Addition  use_carryin=off  use_carryout=off  en=off  latency=1  precision=Full  arith_type=Unsigned  n_bits=16  bin_pt=14  quantization=Truncate  overflow=Wrap  dbl_ovrd=off  use_behavioral_HDL=off  hw_selection=DSP48  pipelined=on  use_rpm=on  block_type=addsub
  dly26 : xbsIndex_r4/Delay  rst=off  infoeditControl=Selection of Reset will increase slice count due to use of real FFs and instead of SRLs  en=off  latency=1  dbl_ovrd=off  reg_retiming=on  block_type=delay
  dly46 : xbsIndex_r4/Delay  rst=off  infoeditControl=Selection of Reset will increase slice count due to use of real FFs and instead of SRLs  en=off  latency=1  dbl_ovrd=off  reg_retiming=on  block_type=delay
  dly50 : xbsIndex_r4/Delay  rst=off  infoeditControl=Selection of Reset will increase slice count due to use of real FFs and instead of SRLs  en=off  latency=1  dbl_ovrd=off  reg_retiming=on  block_type=delay
  sync_delay : xbsIndex_r4/Delay  rst=off  infoeditControl=Selection of Reset will increase slice count due to use of real FFs and instead of SRLs  en=off  latency=6  dbl_ovrd=off  reg_retiming=on  block_type=delay
      settings: block_version=11.4
  sync_out : Outport
  dout : Outport  Port=2
  wires:
  sync/1 -> sync_delay/1
  sync_delay/1 -> sync_out/1
  din1/1 -> addr1/1
  din2/1 -> addr1/2
  din3/1 -> addr2/1
  din4/1 -> addr2/2
  din5/1 -> addr3/1
  din6/1 -> addr3/2
  din7/1 -> addr4/1
  din8/1 -> addr4/2
  din9/1 -> addr5/1
  din10/1 -> addr5/2
  din11/1 -> addr6/1
  din12/1 -> addr6/2
  din13/1 -> addr7/1
  din14/1 -> addr7/2
  din15/1 -> addr8/1
  din16/1 -> addr8/2
  din17/1 -> addr9/1
  din18/1 -> addr9/2
  din19/1 -> addr10/1
  din20/1 -> addr10/2
  din21/1 -> addr11/1
  din22/1 -> addr11/2
  din23/1 -> addr12/1
  din24/1 -> addr12/2
  din25/1 -> addr13/1
  din26/1 -> addr13/2
  din27/1 -> addr14/1
  din28/1 -> addr14/2
  din29/1 -> addr15/1
  din30/1 -> addr15/2
  din31/1 -> addr16/1
  din32/1 -> addr16/2
  din33/1 -> addr17/1
  din34/1 -> addr17/2
  din35/1 -> addr18/1
  din36/1 -> addr18/2
  din37/1 -> addr19/1
  din38/1 -> addr19/2
  din39/1 -> addr20/1
  din40/1 -> addr20/2
  din41/1 -> addr21/1
  din42/1 -> addr21/2
  din43/1 -> addr22/1
  din44/1 -> addr22/2
  din45/1 -> addr23/1
  din46/1 -> addr23/2
  din47/1 -> addr24/1
  din48/1 -> addr24/2
  din49/1 -> addr25/1
  din50/1 -> addr25/2
  din51/1 -> dly26/1
  addr1/1 -> addr27/1
  addr2/1 -> addr27/2
  addr3/1 -> addr28/1
  addr4/1 -> addr28/2
  addr5/1 -> addr29/1
  addr6/1 -> addr29/2
  addr7/1 -> addr30/1
  addr8/1 -> addr30/2
  addr9/1 -> addr31/1
  addr10/1 -> addr31/2
  addr11/1 -> addr32/1
  addr12/1 -> addr32/2
  addr13/1 -> addr33/1
  addr14/1 -> addr33/2
  addr15/1 -> addr34/1
  addr16/1 -> addr34/2
  addr17/1 -> addr35/1
  addr18/1 -> addr35/2
  addr19/1 -> addr36/1
  addr20/1 -> addr36/2
  addr21/1 -> addr37/1
  addr22/1 -> addr37/2
  addr23/1 -> addr38/1
  addr24/1 -> addr38/2
  addr25/1 -> addr39/1
  dly26/1 -> addr39/2
  addr27/1 -> addr40/1
  addr28/1 -> addr40/2
  addr29/1 -> addr41/1
  addr30/1 -> addr41/2
  addr31/1 -> addr42/1
  addr32/1 -> addr42/2
  addr33/1 -> addr43/1
  addr34/1 -> addr43/2
  addr35/1 -> addr44/1
  addr36/1 -> addr44/2
  addr37/1 -> addr45/1
  addr38/1 -> addr45/2
  addr39/1 -> dly46/1
  addr40/1 -> addr47/1
  addr41/1 -> addr47/2
  addr42/1 -> addr48/1
  addr43/1 -> addr48/2
  addr44/1 -> addr49/1
  addr45/1 -> addr49/2
  dly46/1 -> dly50/1
  addr47/1 -> addr51/1
  addr48/1 -> addr51/2
  addr49/1 -> addr52/1
  dly50/1 -> addr52/2
  addr51/1 -> addr53/1
  addr52/1 -> addr53/2
  addr53/1 -> dout/1

== system lo_values_test_v11/dec_fir3/fir_dbl_col1 ==
  real1 : Inport
  imag1 : Inport  Port=2
  real_back1 : Inport  Port=3
  imag_back1 : Inport  Port=4
  fir_dbl_tap1 : Subsystem  AncestorBlock=casper_library_downconverter/fir_dbl_tap  mask(fir_dbl_tap){factor=0.00034504, add_latency=add_latency, mult_latency=mult_latency, coeff_bit_width=coeff_bit_width, coeff_bin_pt=coeff_bin_pt}
      mask prompts: add_latency "Add latency"; mult_latency "Mult latency"; coeff_bit_width "Coefficient bit width"; coeff_bin_pt "Coefficient binary point"
      mask init: same as lo_values_test_v11/dec_fir/fir_dbl_col1/fir_dbl_tap1
      mask Help: eval('xlWeb(''http://casper.berkeley.edu/wiki/Fir_dbl_tap'')')
  real_out1 : Outport
  imag_out1 : Outport  Port=2
  real_back_out1 : Outport  Port=3
  imag_back_out1 : Outport  Port=4
  real_sum : Outport  Port=5
  imag_sum : Outport  Port=6
  wires:
  real1/1 -> fir_dbl_tap1/1(a)
  imag1/1 -> fir_dbl_tap1/2(b)
  real_back1/1 -> fir_dbl_tap1/3(c)
  imag_back1/1 -> fir_dbl_tap1/4(d)
  fir_dbl_tap1/1(a_out) -> real_out1/1
  fir_dbl_tap1/2(b_out) -> imag_out1/1
  fir_dbl_tap1/3(c_out) -> real_back_out1/1
  fir_dbl_tap1/4(d_out) -> imag_back_out1/1
  fir_dbl_tap1/5(real) -> real_sum/1
  fir_dbl_tap1/6(imag) -> imag_sum/1

== system lo_values_test_v11/dec_fir3/fir_dbl_col10 ==
  real1 : Inport
  imag1 : Inport  Port=2
  real_back1 : Inport  Port=3
  imag_back1 : Inport  Port=4
  fir_dbl_tap1 : Subsystem  AncestorBlock=casper_library_downconverter/fir_dbl_tap  mask(fir_dbl_tap){factor=0.0011044, add_latency=add_latency, mult_latency=mult_latency, coeff_bit_width=coeff_bit_width, coeff_bin_pt=coeff_bin_pt}
      mask prompts: add_latency "Add latency"; mult_latency "Mult latency"; coeff_bit_width "Coefficient bit width"; coeff_bin_pt "Coefficient binary point"
      mask init: same as lo_values_test_v11/dec_fir/fir_dbl_col1/fir_dbl_tap1
      mask Help: eval('xlWeb(''http://casper.berkeley.edu/wiki/Fir_dbl_tap'')')
  real_out1 : Outport
  imag_out1 : Outport  Port=2
  real_back_out1 : Outport  Port=3
  imag_back_out1 : Outport  Port=4
  real_sum : Outport  Port=5
  imag_sum : Outport  Port=6
  wires:
  real1/1 -> fir_dbl_tap1/1(a)
  imag1/1 -> fir_dbl_tap1/2(b)
  real_back1/1 -> fir_dbl_tap1/3(c)
  imag_back1/1 -> fir_dbl_tap1/4(d)
  fir_dbl_tap1/1(a_out) -> real_out1/1
  fir_dbl_tap1/2(b_out) -> imag_out1/1
  fir_dbl_tap1/3(c_out) -> real_back_out1/1
  fir_dbl_tap1/4(d_out) -> imag_back_out1/1
  fir_dbl_tap1/5(real) -> real_sum/1
  fir_dbl_tap1/6(imag) -> imag_sum/1

== system lo_values_test_v11/dec_fir3/fir_dbl_col11 ==
  real1 : Inport
  imag1 : Inport  Port=2
  real_back1 : Inport  Port=3
  imag_back1 : Inport  Port=4
  fir_dbl_tap1 : Subsystem  AncestorBlock=casper_library_downconverter/fir_dbl_tap  mask(fir_dbl_tap){factor=0.0012861, add_latency=add_latency, mult_latency=mult_latency, coeff_bit_width=coeff_bit_width, coeff_bin_pt=coeff_bin_pt}
      mask prompts: add_latency "Add latency"; mult_latency "Mult latency"; coeff_bit_width "Coefficient bit width"; coeff_bin_pt "Coefficient binary point"
      mask init: same as lo_values_test_v11/dec_fir/fir_dbl_col1/fir_dbl_tap1
      mask Help: eval('xlWeb(''http://casper.berkeley.edu/wiki/Fir_dbl_tap'')')
  real_out1 : Outport
  imag_out1 : Outport  Port=2
  real_back_out1 : Outport  Port=3
  imag_back_out1 : Outport  Port=4
  real_sum : Outport  Port=5
  imag_sum : Outport  Port=6
  wires:
  real1/1 -> fir_dbl_tap1/1(a)
  imag1/1 -> fir_dbl_tap1/2(b)
  real_back1/1 -> fir_dbl_tap1/3(c)
  imag_back1/1 -> fir_dbl_tap1/4(d)
  fir_dbl_tap1/1(a_out) -> real_out1/1
  fir_dbl_tap1/2(b_out) -> imag_out1/1
  fir_dbl_tap1/3(c_out) -> real_back_out1/1
  fir_dbl_tap1/4(d_out) -> imag_back_out1/1
  fir_dbl_tap1/5(real) -> real_sum/1
  fir_dbl_tap1/6(imag) -> imag_sum/1

== system lo_values_test_v11/dec_fir3/fir_dbl_col12 ==
  real1 : Inport
  imag1 : Inport  Port=2
  real_back1 : Inport  Port=3
  imag_back1 : Inport  Port=4
  fir_dbl_tap1 : Subsystem  AncestorBlock=casper_library_downconverter/fir_dbl_tap  mask(fir_dbl_tap){factor=0.0014864, add_latency=add_latency, mult_latency=mult_latency, coeff_bit_width=coeff_bit_width, coeff_bin_pt=coeff_bin_pt}
      mask prompts: add_latency "Add latency"; mult_latency "Mult latency"; coeff_bit_width "Coefficient bit width"; coeff_bin_pt "Coefficient binary point"
      mask init: same as lo_values_test_v11/dec_fir/fir_dbl_col1/fir_dbl_tap1
      mask Help: eval('xlWeb(''http://casper.berkeley.edu/wiki/Fir_dbl_tap'')')
  real_out1 : Outport
  imag_out1 : Outport  Port=2
  real_back_out1 : Outport  Port=3
  imag_back_out1 : Outport  Port=4
  real_sum : Outport  Port=5
  imag_sum : Outport  Port=6
  wires:
  real1/1 -> fir_dbl_tap1/1(a)
  imag1/1 -> fir_dbl_tap1/2(b)
  real_back1/1 -> fir_dbl_tap1/3(c)
  imag_back1/1 -> fir_dbl_tap1/4(d)
  fir_dbl_tap1/1(a_out) -> real_out1/1
  fir_dbl_tap1/2(b_out) -> imag_out1/1
  fir_dbl_tap1/3(c_out) -> real_back_out1/1
  fir_dbl_tap1/4(d_out) -> imag_back_out1/1
  fir_dbl_tap1/5(real) -> real_sum/1
  fir_dbl_tap1/6(imag) -> imag_sum/1

== system lo_values_test_v11/dec_fir3/fir_dbl_col13 ==
  real1 : Inport
  imag1 : Inport  Port=2
  real_back1 : Inport  Port=3
  imag_back1 : Inport  Port=4
  fir_dbl_tap1 : Subsystem  AncestorBlock=casper_library_downconverter/fir_dbl_tap  mask(fir_dbl_tap){factor=0.0017056, add_latency=add_latency, mult_latency=mult_latency, coeff_bit_width=coeff_bit_width, coeff_bin_pt=coeff_bin_pt}
      mask prompts: add_latency "Add latency"; mult_latency "Mult latency"; coeff_bit_width "Coefficient bit width"; coeff_bin_pt "Coefficient binary point"
      mask init: same as lo_values_test_v11/dec_fir/fir_dbl_col1/fir_dbl_tap1
      mask Help: eval('xlWeb(''http://casper.berkeley.edu/wiki/Fir_dbl_tap'')')
  real_out1 : Outport
  imag_out1 : Outport  Port=2
  real_back_out1 : Outport  Port=3
  imag_back_out1 : Outport  Port=4
  real_sum : Outport  Port=5
  imag_sum : Outport  Port=6
  wires:
  real1/1 -> fir_dbl_tap1/1(a)
  imag1/1 -> fir_dbl_tap1/2(b)
  real_back1/1 -> fir_dbl_tap1/3(c)
  imag_back1/1 -> fir_dbl_tap1/4(d)
  fir_dbl_tap1/1(a_out) -> real_out1/1
  fir_dbl_tap1/2(b_out) -> imag_out1/1
  fir_dbl_tap1/3(c_out) -> real_back_out1/1
  fir_dbl_tap1/4(d_out) -> imag_back_out1/1
  fir_dbl_tap1/5(real) -> real_sum/1
  fir_dbl_tap1/6(imag) -> imag_sum/1

== system lo_values_test_v11/dec_fir3/fir_dbl_col14 ==
  real1 : Inport
  imag1 : Inport  Port=2
  real_back1 : Inport  Port=3
  imag_back1 : Inport  Port=4
  fir_dbl_tap1 : Subsystem  AncestorBlock=casper_library_downconverter/fir_dbl_tap  mask(fir_dbl_tap){factor=0.0019439, add_latency=add_latency, mult_latency=mult_latency, coeff_bit_width=coeff_bit_width, coeff_bin_pt=coeff_bin_pt}
      mask prompts: add_latency "Add latency"; mult_latency "Mult latency"; coeff_bit_width "Coefficient bit width"; coeff_bin_pt "Coefficient binary point"
      mask init: same as lo_values_test_v11/dec_fir/fir_dbl_col1/fir_dbl_tap1
      mask Help: eval('xlWeb(''http://casper.berkeley.edu/wiki/Fir_dbl_tap'')')
  real_out1 : Outport
  imag_out1 : Outport  Port=2
  real_back_out1 : Outport  Port=3
  imag_back_out1 : Outport  Port=4
  real_sum : Outport  Port=5
  imag_sum : Outport  Port=6
  wires:
  real1/1 -> fir_dbl_tap1/1(a)
  imag1/1 -> fir_dbl_tap1/2(b)
  real_back1/1 -> fir_dbl_tap1/3(c)
  imag_back1/1 -> fir_dbl_tap1/4(d)
  fir_dbl_tap1/1(a_out) -> real_out1/1
  fir_dbl_tap1/2(b_out) -> imag_out1/1
  fir_dbl_tap1/3(c_out) -> real_back_out1/1
  fir_dbl_tap1/4(d_out) -> imag_back_out1/1
  fir_dbl_tap1/5(real) -> real_sum/1
  fir_dbl_tap1/6(imag) -> imag_sum/1

== system lo_values_test_v11/dec_fir3/fir_dbl_col15 ==
  real1 : Inport
  imag1 : Inport  Port=2
  real_back1 : Inport  Port=3
  imag_back1 : Inport  Port=4
  fir_dbl_tap1 : Subsystem  AncestorBlock=casper_library_downconverter/fir_dbl_tap  mask(fir_dbl_tap){factor=0.0022021, add_latency=add_latency, mult_latency=mult_latency, coeff_bit_width=coeff_bit_width, coeff_bin_pt=coeff_bin_pt}
      mask prompts: add_latency "Add latency"; mult_latency "Mult latency"; coeff_bit_width "Coefficient bit width"; coeff_bin_pt "Coefficient binary point"
      mask init: same as lo_values_test_v11/dec_fir/fir_dbl_col1/fir_dbl_tap1
      mask Help: eval('xlWeb(''http://casper.berkeley.edu/wiki/Fir_dbl_tap'')')
  real_out1 : Outport
  imag_out1 : Outport  Port=2
  real_back_out1 : Outport  Port=3
  imag_back_out1 : Outport  Port=4
  real_sum : Outport  Port=5
  imag_sum : Outport  Port=6
  wires:
  real1/1 -> fir_dbl_tap1/1(a)
  imag1/1 -> fir_dbl_tap1/2(b)
  real_back1/1 -> fir_dbl_tap1/3(c)
  imag_back1/1 -> fir_dbl_tap1/4(d)
  fir_dbl_tap1/1(a_out) -> real_out1/1
  fir_dbl_tap1/2(b_out) -> imag_out1/1
  fir_dbl_tap1/3(c_out) -> real_back_out1/1
  fir_dbl_tap1/4(d_out) -> imag_back_out1/1
  fir_dbl_tap1/5(real) -> real_sum/1
  fir_dbl_tap1/6(imag) -> imag_sum/1

== system lo_values_test_v11/dec_fir3/fir_dbl_col16 ==
  real1 : Inport
  imag1 : Inport  Port=2
  real_back1 : Inport  Port=3
  imag_back1 : Inport  Port=4
  fir_dbl_tap1 : Subsystem  AncestorBlock=casper_library_downconverter/fir_dbl_tap  mask(fir_dbl_tap){factor=0.0024799, add_latency=add_latency, mult_latency=mult_latency, coeff_bit_width=coeff_bit_width, coeff_bin_pt=coeff_bin_pt}
      mask prompts: add_latency "Add latency"; mult_latency "Mult latency"; coeff_bit_width "Coefficient bit width"; coeff_bin_pt "Coefficient binary point"
      mask init: same as lo_values_test_v11/dec_fir/fir_dbl_col1/fir_dbl_tap1
      mask Help: eval('xlWeb(''http://casper.berkeley.edu/wiki/Fir_dbl_tap'')')
  real_out1 : Outport
  imag_out1 : Outport  Port=2
  real_back_out1 : Outport  Port=3
  imag_back_out1 : Outport  Port=4
  real_sum : Outport  Port=5
  imag_sum : Outport  Port=6
  wires:
  real1/1 -> fir_dbl_tap1/1(a)
  imag1/1 -> fir_dbl_tap1/2(b)
  real_back1/1 -> fir_dbl_tap1/3(c)
  imag_back1/1 -> fir_dbl_tap1/4(d)
  fir_dbl_tap1/1(a_out) -> real_out1/1
  fir_dbl_tap1/2(b_out) -> imag_out1/1
  fir_dbl_tap1/3(c_out) -> real_back_out1/1
  fir_dbl_tap1/4(d_out) -> imag_back_out1/1
  fir_dbl_tap1/5(real) -> real_sum/1
  fir_dbl_tap1/6(imag) -> imag_sum/1

== system lo_values_test_v11/dec_fir3/fir_dbl_col17 ==
  real1 : Inport
  imag1 : Inport  Port=2
  real_back1 : Inport  Port=3
  imag_back1 : Inport  Port=4
  fir_dbl_tap1 : Subsystem  AncestorBlock=casper_library_downconverter/fir_dbl_tap  mask(fir_dbl_tap){factor=0.0027778, add_latency=add_latency, mult_latency=mult_latency, coeff_bit_width=coeff_bit_width, coeff_bin_pt=coeff_bin_pt}
      mask prompts: add_latency "Add latency"; mult_latency "Mult latency"; coeff_bit_width "Coefficient bit width"; coeff_bin_pt "Coefficient binary point"
      mask init: same as lo_values_test_v11/dec_fir/fir_dbl_col1/fir_dbl_tap1
      mask Help: eval('xlWeb(''http://casper.berkeley.edu/wiki/Fir_dbl_tap'')')
  real_out1 : Outport
  imag_out1 : Outport  Port=2
  real_back_out1 : Outport  Port=3
  imag_back_out1 : Outport  Port=4
  real_sum : Outport  Port=5
  imag_sum : Outport  Port=6
  wires:
  real1/1 -> fir_dbl_tap1/1(a)
  imag1/1 -> fir_dbl_tap1/2(b)
  real_back1/1 -> fir_dbl_tap1/3(c)
  imag_back1/1 -> fir_dbl_tap1/4(d)
  fir_dbl_tap1/1(a_out) -> real_out1/1
  fir_dbl_tap1/2(b_out) -> imag_out1/1
  fir_dbl_tap1/3(c_out) -> real_back_out1/1
  fir_dbl_tap1/4(d_out) -> imag_back_out1/1
  fir_dbl_tap1/5(real) -> real_sum/1
  fir_dbl_tap1/6(imag) -> imag_sum/1

== system lo_values_test_v11/dec_fir3/fir_dbl_col18 ==
  real1 : Inport
  imag1 : Inport  Port=2
  real_back1 : Inport  Port=3
  imag_back1 : Inport  Port=4
  fir_dbl_tap1 : Subsystem  AncestorBlock=casper_library_downconverter/fir_dbl_tap  mask(fir_dbl_tap){factor=0.0030952, add_latency=add_latency, mult_latency=mult_latency, coeff_bit_width=coeff_bit_width, coeff_bin_pt=coeff_bin_pt}
      mask prompts: add_latency "Add latency"; mult_latency "Mult latency"; coeff_bit_width "Coefficient bit width"; coeff_bin_pt "Coefficient binary point"
      mask init: same as lo_values_test_v11/dec_fir/fir_dbl_col1/fir_dbl_tap1
      mask Help: eval('xlWeb(''http://casper.berkeley.edu/wiki/Fir_dbl_tap'')')
  real_out1 : Outport
  imag_out1 : Outport  Port=2
  real_back_out1 : Outport  Port=3
  imag_back_out1 : Outport  Port=4
  real_sum : Outport  Port=5
  imag_sum : Outport  Port=6
  wires:
  real1/1 -> fir_dbl_tap1/1(a)
  imag1/1 -> fir_dbl_tap1/2(b)
  real_back1/1 -> fir_dbl_tap1/3(c)
  imag_back1/1 -> fir_dbl_tap1/4(d)
  fir_dbl_tap1/1(a_out) -> real_out1/1
  fir_dbl_tap1/2(b_out) -> imag_out1/1
  fir_dbl_tap1/3(c_out) -> real_back_out1/1
  fir_dbl_tap1/4(d_out) -> imag_back_out1/1
  fir_dbl_tap1/5(real) -> real_sum/1
  fir_dbl_tap1/6(imag) -> imag_sum/1
